simulink model "E_7"  (R2017a)
settings: Solver=VariableStepAuto  StartTime=0.0  StopTime=50  RelTol=1e-3
settings Model: Creator=Mat Haskell  LastModifiedBy=Mat Haskell

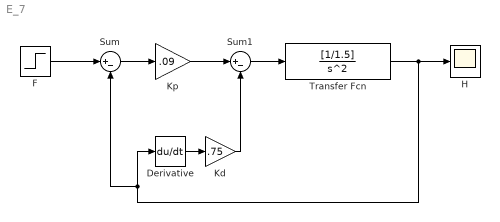
== system E_7 ==
  Derivative : Derivative
  "F " : Step  SampleTime=0
  "H " : Scope
  "Kd " : Gain  Gain=.75
  Kp : Gain  Gain=.09
  Sum : Sum  Inputs=|+-
  Sum1 : Sum  Inputs=|+-
  Transfer Fcn : TransferFcn  Numerator=[1/1.5]  Denominator=[1 0 0]
  wires:
  "F "/1 -> Sum/1
  Sum/1 -> Kp/1
  Kp/1 -> Sum1/1
  Sum1/1 -> Transfer Fcn/1
  Transfer Fcn/1 -> Sum/2, Derivative/1, "H "/1
  Derivative/1 -> "Kd "/1
  "Kd "/1 -> Sum1/2
